simulink model "line_choices_snt"  (R2025b)
settings: Solver=ode45  StartTime=0.0  StopTime=10.0  RelTol=1e-3  EnableMultiTasking=on
values from neighbouring files (symbols this model uses):
  ft2km = 0.0003048    [IEEE_123_data.m]    (also in IEEE_123_data_fault.m)
undefined symbols (not defined in the file or in its folder): C_1, find_system, L_1, R_1
libraries: fl_lib x156, nesl_utility x24
(part 2 of 2)

== system line_choices_snt/T2sscT/OLTC ==
  Electrical Reference : fl_lib/Electrical/Electrical Elements/Electrical Reference
  Electrical Reference1 : fl_lib/Electrical/Electrical Elements/Electrical Reference
  TA : Subsystem
  TB : Subsystem
  A : PMIOPort  Tag=PMCPort  Side=Left
  B : PMIOPort  Tag=PMCPort  Port=2  Side=Left
  a : PMIOPort  Tag=PMCPort  Port=3  Side=Right
  b : PMIOPort  Tag=PMCPort  Port=4  Side=Right
  connections:
  Electrical Reference1/LConn1 -- TB/RConn2 -- TA/RConn2
  TA/RConn1 -- a/RConn1
  TA/LConn1 -- A/RConn1
  TB/LConn1 -- B/RConn1
  TB/RConn1 -- b/RConn1
  Electrical Reference/LConn1 -- TB/LConn2 -- TA/LConn2

== system line_choices_snt/T2sscT/Pi-Section Line ==
  Array Connection{,1..3} (4 alike) : SimscapeArrayConnection
  Electrical Reference : fl_lib/Electrical/Electrical Elements/Electrical Reference
  Electrical Reference1 : fl_lib/Electrical/Electrical Elements/Electrical Reference
  Mutual C1 : SimscapeComponentBlock  SourceFile=multi_coupled_C  ComponentPath=multi_coupled_C  ComponentVariants="[\"multi_coupled_C\"]"  ComponentVariantNames="[\"multi_coupled_C\"]"  ClassName=multi_coupled_C  SchemaVersion=1  noph=2  C=C F
      settings: CopyFcn=simscape.sscblock.internal.componentBlockCallback(gcbh,'COPY')  PreCopyFcn=simscape.sscblock.internal.componentBlockCallback(gcbh,'PRECOPY')  PreDeleteFcn=simscape.sscblock.internal.componentBlockCallback(gcbh,'PREDELETE')  InternalSimscapePortConfiguration="{\"Bottom\":[],\"Left\":[{\"id\":\"p\",\"label\":\"p\",\"type\":\"foundation.electrical.electrical\"}],\"Right\":[{\"id\":\"n\",\"label\":\"n\",\"type\":\"foundation.electrical.electrical\"}],\"Top\":[]}"
      mask Type: Multi-Phase Coupled C
  Mutual C2 : SimscapeComponentBlock  SourceFile=multi_coupled_C  ComponentPath=multi_coupled_C  ComponentVariants="[\"multi_coupled_C\"]"  ComponentVariantNames="[\"multi_coupled_C\"]"  ClassName=multi_coupled_C  SchemaVersion=1  noph=2  C=C F
      settings: CopyFcn=simscape.sscblock.internal.componentBlockCallback(gcbh,'COPY')  PreCopyFcn=simscape.sscblock.internal.componentBlockCallback(gcbh,'PRECOPY')  PreDeleteFcn=simscape.sscblock.internal.componentBlockCallback(gcbh,'PREDELETE')  InternalSimscapePortConfiguration="{\"Bottom\":[],\"Left\":[{\"id\":\"p\",\"label\":\"p\",\"type\":\"foundation.electrical.electrical\"}],\"Right\":[{\"id\":\"n\",\"label\":\"n\",\"type\":\"foundation.electrical.electrical\"}],\"Top\":[]}"
      mask Type: Multi-Phase Coupled C
  Mutual RL : SimscapeComponentBlock  SourceFile=multi_coupled_RL  ComponentPath=multi_coupled_RL  ComponentVariants="[\"multi_coupled_RL\"]"  ComponentVariantNames="[\"multi_coupled_RL\"]"  ClassName=multi_coupled_RL  SchemaVersion=1  noph=2  R=R Ohm  L=L H
      settings: CopyFcn=simscape.sscblock.internal.componentBlockCallback(gcbh,'COPY')  PreCopyFcn=simscape.sscblock.internal.componentBlockCallback(gcbh,'PRECOPY')  PreDeleteFcn=simscape.sscblock.internal.componentBlockCallback(gcbh,'PREDELETE')  InternalSimscapePortConfiguration="{\"Bottom\":[],\"Left\":[{\"id\":\"p\",\"label\":\"p\",\"type\":\"foundation.electrical.electrical\"}],\"Right\":[{\"id\":\"n\",\"label\":\"n\",\"type\":\"foundation.electrical.electrical\"}],\"Top\":[]}"
      mask Type: Multi-Phase Coupled RL
  PS-Simulink Converter : nesl_utility/PS-Simulink Converter  PhysicalDomain=network_engine_domain  SubClassName=ps_output  LeftPortType=input  RightPortType=output  PseudoPeriodic=off  Frequencies=[]  VectorFormat=inherit  Unit=inherit  AffineConversion=off
  Simscape Component : SimscapeComponentBlock  SourceFile=multi_current  ComponentPath=multi_current  ComponentVariants="[\"multi_current\"]"  ComponentVariantNames="[\"multi_current\"]"  ClassName=multi_current  SchemaVersion=1  noph=2
      settings: CopyFcn=simscape.sscblock.internal.componentBlockCallback(gcbh,'COPY')  PreCopyFcn=simscape.sscblock.internal.componentBlockCallback(gcbh,'PRECOPY')  PreDeleteFcn=simscape.sscblock.internal.componentBlockCallback(gcbh,'PREDELETE')  InternalSimscapePortConfiguration="{\"Bottom\":[],\"Left\":[{\"id\":\"p\",\"label\":\"+\",\"type\":\"foundation.electrical.electrical\"}],\"Right\":[{\"id\":\"I\",\"label\":\"I\",\"type\":\"output\"},{\"id\":\"n\",\"label\":\"-\",\"type\":\"foundation.electrical.electrical\"}],\"Top\":[]}"
      mask Type: Multi-Phase Current Sensor
  A : PMIOPort  Side=Left
  B : PMIOPort  Port=2  Side=Left
  a : PMIOPort  Port=3  Side=Right
  b : PMIOPort  Port=4  Side=Right
  Imeas : Outport
  wires:
  PS-Simulink Converter/1 -> Imeas/1
  connections:
  Mutual RL/RConn1 -- Array Connection1/RConn1 -- Mutual C2/LConn1
  Mutual C1/LConn1 -- Simscape Component/RConn2 -- Mutual RL/LConn1
  PS-Simulink Converter/LConn1 -- Simscape Component/RConn1
  Array Connection/RConn1 -- Simscape Component/LConn1
  A/RConn1 -- Array Connection/LConn1
  B/RConn1 -- Array Connection/LConn2
  a/RConn1 -- Array Connection1/LConn1
  b/RConn1 -- Array Connection1/LConn2
  Array Connection2/RConn1 -- Mutual C1/RConn1
  Array Connection3/RConn1 -- Mutual C2/RConn1
  Array Connection2/LConn1 -- Electrical Reference/LConn1 -- Array Connection2/LConn2
  Array Connection3/LConn1 -- Electrical Reference1/LConn1 -- Array Connection3/LConn2

== system line_choices_snt/T2sscTf/OLTC ==
  Electrical Reference : fl_lib/Electrical/Electrical Elements/Electrical Reference
  Electrical Reference1 : fl_lib/Electrical/Electrical Elements/Electrical Reference
  TA : Subsystem
  TB : Subsystem
  A : PMIOPort  Tag=PMCPort  Side=Left
  B : PMIOPort  Tag=PMCPort  Port=2  Side=Left
  a : PMIOPort  Tag=PMCPort  Port=3  Side=Right
  b : PMIOPort  Tag=PMCPort  Port=4  Side=Right
  connections:
  TA/LConn2 -- TB/LConn2 -- Electrical Reference/LConn1
  TB/RConn1 -- b/RConn1
  TB/LConn1 -- B/RConn1
  TA/LConn1 -- A/RConn1
  TA/RConn1 -- a/RConn1
  TA/RConn2 -- TB/RConn2 -- Electrical Reference1/LConn1

== system line_choices_snt/T2sscTf/Pi-Section Line ==
  Array Connection{,1..3} (4 alike) : SimscapeArrayConnection
  Electrical Reference : fl_lib/Electrical/Electrical Elements/Electrical Reference
  Electrical Reference1 : fl_lib/Electrical/Electrical Elements/Electrical Reference
  Mutual C1 : SimscapeComponentBlock  SourceFile=multi_coupled_C  ComponentPath=multi_coupled_C  ComponentVariants="[\"multi_coupled_C\"]"  ComponentVariantNames="[\"multi_coupled_C\"]"  ClassName=multi_coupled_C  SchemaVersion=1  noph=2  C=C F
      settings: CopyFcn=simscape.sscblock.internal.componentBlockCallback(gcbh,'COPY')  PreCopyFcn=simscape.sscblock.internal.componentBlockCallback(gcbh,'PRECOPY')  PreDeleteFcn=simscape.sscblock.internal.componentBlockCallback(gcbh,'PREDELETE')  InternalSimscapePortConfiguration="{\"Bottom\":[],\"Left\":[{\"id\":\"p\",\"label\":\"p\",\"type\":\"foundation.electrical.electrical\"}],\"Right\":[{\"id\":\"n\",\"label\":\"n\",\"type\":\"foundation.electrical.electrical\"}],\"Top\":[]}"
      mask Type: Multi-Phase Coupled C
  Mutual C2 : SimscapeComponentBlock  SourceFile=multi_coupled_C  ComponentPath=multi_coupled_C  ComponentVariants="[\"multi_coupled_C\"]"  ComponentVariantNames="[\"multi_coupled_C\"]"  ClassName=multi_coupled_C  SchemaVersion=1  noph=2  C=C F
      settings: CopyFcn=simscape.sscblock.internal.componentBlockCallback(gcbh,'COPY')  PreCopyFcn=simscape.sscblock.internal.componentBlockCallback(gcbh,'PRECOPY')  PreDeleteFcn=simscape.sscblock.internal.componentBlockCallback(gcbh,'PREDELETE')  InternalSimscapePortConfiguration="{\"Bottom\":[],\"Left\":[{\"id\":\"p\",\"label\":\"p\",\"type\":\"foundation.electrical.electrical\"}],\"Right\":[{\"id\":\"n\",\"label\":\"n\",\"type\":\"foundation.electrical.electrical\"}],\"Top\":[]}"
      mask Type: Multi-Phase Coupled C
  Mutual RL : SimscapeComponentBlock  SourceFile=multi_coupled_RL  ComponentPath=multi_coupled_RL  ComponentVariants="[\"multi_coupled_RL\"]"  ComponentVariantNames="[\"multi_coupled_RL\"]"  ClassName=multi_coupled_RL  SchemaVersion=1  noph=2  R=R Ohm  L=L H
      settings: CopyFcn=simscape.sscblock.internal.componentBlockCallback(gcbh,'COPY')  PreCopyFcn=simscape.sscblock.internal.componentBlockCallback(gcbh,'PRECOPY')  PreDeleteFcn=simscape.sscblock.internal.componentBlockCallback(gcbh,'PREDELETE')  InternalSimscapePortConfiguration="{\"Bottom\":[],\"Left\":[{\"id\":\"p\",\"label\":\"p\",\"type\":\"foundation.electrical.electrical\"}],\"Right\":[{\"id\":\"n\",\"label\":\"n\",\"type\":\"foundation.electrical.electrical\"}],\"Top\":[]}"
      mask Type: Multi-Phase Coupled RL
  PS-Simulink Converter : nesl_utility/PS-Simulink Converter  PhysicalDomain=network_engine_domain  SubClassName=ps_output  LeftPortType=input  RightPortType=output  PseudoPeriodic=off  Frequencies=[]  VectorFormat=inherit  Unit=inherit  AffineConversion=off
  Simscape Component : SimscapeComponentBlock  SourceFile=multi_current  ComponentPath=multi_current  ComponentVariants="[\"multi_current\"]"  ComponentVariantNames="[\"multi_current\"]"  ClassName=multi_current  SchemaVersion=1  noph=2
      settings: CopyFcn=simscape.sscblock.internal.componentBlockCallback(gcbh,'COPY')  PreCopyFcn=simscape.sscblock.internal.componentBlockCallback(gcbh,'PRECOPY')  PreDeleteFcn=simscape.sscblock.internal.componentBlockCallback(gcbh,'PREDELETE')  InternalSimscapePortConfiguration="{\"Bottom\":[],\"Left\":[{\"id\":\"p\",\"label\":\"+\",\"type\":\"foundation.electrical.electrical\"}],\"Right\":[{\"id\":\"I\",\"label\":\"I\",\"type\":\"output\"},{\"id\":\"n\",\"label\":\"-\",\"type\":\"foundation.electrical.electrical\"}],\"Top\":[]}"
      mask Type: Multi-Phase Current Sensor
  A : PMIOPort  Side=Left
  B : PMIOPort  Port=2  Side=Left
  a : PMIOPort  Port=3  Side=Right
  b : PMIOPort  Port=4  Side=Right
  Imeas : Outport
  wires:
  PS-Simulink Converter/1 -> Imeas/1
  connections:
  Array Connection3/LConn2 -- Electrical Reference1/LConn1 -- Array Connection3/LConn1
  Array Connection2/LConn2 -- Electrical Reference/LConn1 -- Array Connection2/LConn1
  Array Connection3/RConn1 -- Mutual C2/RConn1
  Array Connection2/RConn1 -- Mutual C1/RConn1
  b/RConn1 -- Array Connection1/LConn2
  a/RConn1 -- Array Connection1/LConn1
  B/RConn1 -- Array Connection/LConn2
  A/RConn1 -- Array Connection/LConn1
  Array Connection/RConn1 -- Simscape Component/LConn1
  PS-Simulink Converter/LConn1 -- Simscape Component/RConn1
  Mutual RL/LConn1 -- Simscape Component/RConn2 -- Mutual C1/LConn1
  Mutual C2/LConn1 -- Array Connection1/RConn1 -- Mutual RL/RConn1

== system line_choices_snt/T3sscT/OLTC ==
  Electrical Reference : fl_lib/Electrical/Electrical Elements/Electrical Reference
  Electrical Reference1 : fl_lib/Electrical/Electrical Elements/Electrical Reference
  TA : Subsystem
  TB : Subsystem
  TC : Subsystem
  A : PMIOPort  Tag=PMCPort  Side=Left
  B : PMIOPort  Tag=PMCPort  Port=2  Side=Left
  C : PMIOPort  Tag=PMCPort  Port=3  Side=Left
  a : PMIOPort  Tag=PMCPort  Port=4  Side=Right
  b : PMIOPort  Tag=PMCPort  Port=5  Side=Right
  c : PMIOPort  Tag=PMCPort  Port=6  Side=Right
  connections:
  TA/RConn1 -- a/RConn1
  TA/LConn1 -- A/RConn1
  TB/LConn1 -- B/RConn1
  TB/RConn1 -- b/RConn1
  TC/LConn1 -- C/RConn1
  TC/RConn1 -- c/RConn1
  TB/RConn2 -- TA/RConn2 -- TC/RConn2 -- Electrical Reference1/LConn1
  TB/LConn2 -- TA/LConn2 -- TC/LConn2 -- Electrical Reference/LConn1

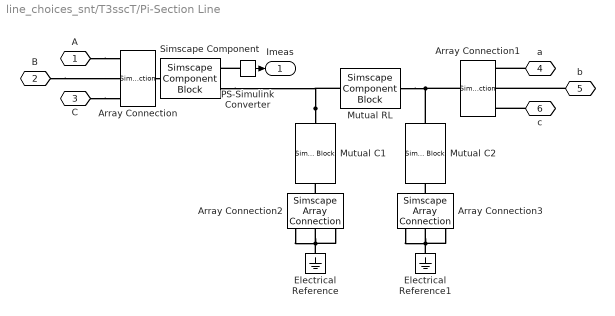
== system line_choices_snt/T3sscT/Pi-Section Line ==
  Array Connection{,1..3} (4 alike) : SimscapeArrayConnection  NumScalarElements=3
  Electrical Reference : fl_lib/Electrical/Electrical Elements/Electrical Reference
  Electrical Reference1 : fl_lib/Electrical/Electrical Elements/Electrical Reference
  Mutual C1 : SimscapeComponentBlock  SourceFile=multi_coupled_C  ComponentPath=multi_coupled_C  ComponentVariants="[\"multi_coupled_C\"]"  ComponentVariantNames="[\"multi_coupled_C\"]"  ClassName=multi_coupled_C  SchemaVersion=1  noph=3  C=C F
      settings: CopyFcn=simscape.sscblock.internal.componentBlockCallback(gcbh,'COPY')  PreCopyFcn=simscape.sscblock.internal.componentBlockCallback(gcbh,'PRECOPY')  PreDeleteFcn=simscape.sscblock.internal.componentBlockCallback(gcbh,'PREDELETE')  InternalSimscapePortConfiguration="{\"Bottom\":[],\"Left\":[{\"id\":\"p\",\"label\":\"p\",\"type\":\"foundation.electrical.electrical\"}],\"Right\":[{\"id\":\"n\",\"label\":\"n\",\"type\":\"foundation.electrical.electrical\"}],\"Top\":[]}"
      mask Type: Multi-Phase Coupled C
  Mutual C2 : SimscapeComponentBlock  SourceFile=multi_coupled_C  ComponentPath=multi_coupled_C  ComponentVariants="[\"multi_coupled_C\"]"  ComponentVariantNames="[\"multi_coupled_C\"]"  ClassName=multi_coupled_C  SchemaVersion=1  noph=3  C=C F
      settings: CopyFcn=simscape.sscblock.internal.componentBlockCallback(gcbh,'COPY')  PreCopyFcn=simscape.sscblock.internal.componentBlockCallback(gcbh,'PRECOPY')  PreDeleteFcn=simscape.sscblock.internal.componentBlockCallback(gcbh,'PREDELETE')  InternalSimscapePortConfiguration="{\"Bottom\":[],\"Left\":[{\"id\":\"p\",\"label\":\"p\",\"type\":\"foundation.electrical.electrical\"}],\"Right\":[{\"id\":\"n\",\"label\":\"n\",\"type\":\"foundation.electrical.electrical\"}],\"Top\":[]}"
      mask Type: Multi-Phase Coupled C
  Mutual RL : SimscapeComponentBlock  SourceFile=multi_coupled_RL  ComponentPath=multi_coupled_RL  ComponentVariants="[\"multi_coupled_RL\"]"  ComponentVariantNames="[\"multi_coupled_RL\"]"  ClassName=multi_coupled_RL  SchemaVersion=1  noph=3  R=R Ohm  L=L H
      settings: CopyFcn=simscape.sscblock.internal.componentBlockCallback(gcbh,'COPY')  PreCopyFcn=simscape.sscblock.internal.componentBlockCallback(gcbh,'PRECOPY')  PreDeleteFcn=simscape.sscblock.internal.componentBlockCallback(gcbh,'PREDELETE')  InternalSimscapePortConfiguration="{\"Bottom\":[],\"Left\":[{\"id\":\"p\",\"label\":\"p\",\"type\":\"foundation.electrical.electrical\"}],\"Right\":[{\"id\":\"n\",\"label\":\"n\",\"type\":\"foundation.electrical.electrical\"}],\"Top\":[]}"
      mask Type: Multi-Phase Coupled RL
  PS-Simulink Converter : nesl_utility/PS-Simulink Converter  PhysicalDomain=network_engine_domain  SubClassName=ps_output  LeftPortType=input  RightPortType=output  PseudoPeriodic=off  Frequencies=[]  VectorFormat=inherit  Unit=inherit  AffineConversion=off
  Simscape Component : SimscapeComponentBlock  SourceFile=multi_current  ComponentPath=multi_current  ComponentVariants="[\"multi_current\"]"  ComponentVariantNames="[\"multi_current\"]"  ClassName=multi_current  SchemaVersion=1  noph=3
      settings: CopyFcn=simscape.sscblock.internal.componentBlockCallback(gcbh,'COPY')  PreCopyFcn=simscape.sscblock.internal.componentBlockCallback(gcbh,'PRECOPY')  PreDeleteFcn=simscape.sscblock.internal.componentBlockCallback(gcbh,'PREDELETE')  InternalSimscapePortConfiguration="{\"Bottom\":[],\"Left\":[{\"id\":\"p\",\"label\":\"+\",\"type\":\"foundation.electrical.electrical\"}],\"Right\":[{\"id\":\"I\",\"label\":\"I\",\"type\":\"output\"},{\"id\":\"n\",\"label\":\"-\",\"type\":\"foundation.electrical.electrical\"}],\"Top\":[]}"
      mask Type: Multi-Phase Current Sensor
  A : PMIOPort  Side=Left
  B : PMIOPort  Port=2  Side=Left
  C : PMIOPort  Port=3  Side=Left
  a : PMIOPort  Port=4  Side=Right
  b : PMIOPort  Port=5  Side=Right
  c : PMIOPort  Port=6  Side=Right
  Imeas : Outport
  wires:
  PS-Simulink Converter/1 -> Imeas/1
  connections:
  Array Connection2/LConn2 -- Array Connection2/LConn3 -- Array Connection2/LConn1 -- Electrical Reference/LConn1
  Mutual RL/RConn1 -- Array Connection1/RConn1 -- Mutual C2/LConn1
  Mutual C1/LConn1 -- Simscape Component/RConn2 -- Mutual RL/LConn1
  Array Connection3/LConn1 -- Array Connection3/LConn2 -- Array Connection3/LConn3 -- Electrical Reference1/LConn1
  Array Connection2/RConn1 -- Mutual C1/RConn1
  Array Connection/RConn1 -- Simscape Component/LConn1
  PS-Simulink Converter/LConn1 -- Simscape Component/RConn1
  Array Connection3/RConn1 -- Mutual C2/RConn1
  A/RConn1 -- Array Connection/LConn1
  B/RConn1 -- Array Connection/LConn2
  C/RConn1 -- Array Connection/LConn3
  a/RConn1 -- Array Connection1/LConn1
  b/RConn1 -- Array Connection1/LConn2
  c/RConn1 -- Array Connection1/LConn3

== system line_choices_snt/T3sscTf/OLTC ==
  Electrical Reference : fl_lib/Electrical/Electrical Elements/Electrical Reference
  Electrical Reference1 : fl_lib/Electrical/Electrical Elements/Electrical Reference
  TA : Subsystem
  TB : Subsystem
  TC : Subsystem
  A : PMIOPort  Tag=PMCPort  Side=Left
  B : PMIOPort  Tag=PMCPort  Port=2  Side=Left
  C : PMIOPort  Tag=PMCPort  Port=3  Side=Left
  a : PMIOPort  Tag=PMCPort  Port=4  Side=Right
  b : PMIOPort  Tag=PMCPort  Port=5  Side=Right
  c : PMIOPort  Tag=PMCPort  Port=6  Side=Right
  connections:
  Electrical Reference/LConn1 -- TC/LConn2 -- TA/LConn2 -- TB/LConn2
  Electrical Reference1/LConn1 -- TC/RConn2 -- TA/RConn2 -- TB/RConn2
  TC/RConn1 -- c/RConn1
  TC/LConn1 -- C/RConn1
  TB/RConn1 -- b/RConn1
  TB/LConn1 -- B/RConn1
  TA/LConn1 -- A/RConn1
  TA/RConn1 -- a/RConn1

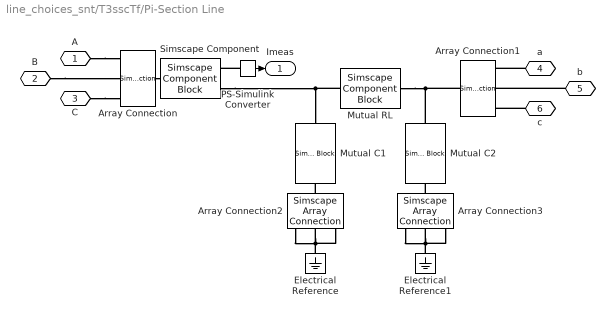
== system line_choices_snt/T3sscTf/Pi-Section Line ==
  Array Connection{,1..3} (4 alike) : SimscapeArrayConnection  NumScalarElements=3
  Electrical Reference : fl_lib/Electrical/Electrical Elements/Electrical Reference
  Electrical Reference1 : fl_lib/Electrical/Electrical Elements/Electrical Reference
  Mutual C1 : SimscapeComponentBlock  SourceFile=multi_coupled_C  ComponentPath=multi_coupled_C  ComponentVariants="[\"multi_coupled_C\"]"  ComponentVariantNames="[\"multi_coupled_C\"]"  ClassName=multi_coupled_C  SchemaVersion=1  noph=3  C=C F
      settings: CopyFcn=simscape.sscblock.internal.componentBlockCallback(gcbh,'COPY')  PreCopyFcn=simscape.sscblock.internal.componentBlockCallback(gcbh,'PRECOPY')  PreDeleteFcn=simscape.sscblock.internal.componentBlockCallback(gcbh,'PREDELETE')  InternalSimscapePortConfiguration="{\"Bottom\":[],\"Left\":[{\"id\":\"p\",\"label\":\"p\",\"type\":\"foundation.electrical.electrical\"}],\"Right\":[{\"id\":\"n\",\"label\":\"n\",\"type\":\"foundation.electrical.electrical\"}],\"Top\":[]}"
      mask Type: Multi-Phase Coupled C
  Mutual C2 : SimscapeComponentBlock  SourceFile=multi_coupled_C  ComponentPath=multi_coupled_C  ComponentVariants="[\"multi_coupled_C\"]"  ComponentVariantNames="[\"multi_coupled_C\"]"  ClassName=multi_coupled_C  SchemaVersion=1  noph=3  C=C F
      settings: CopyFcn=simscape.sscblock.internal.componentBlockCallback(gcbh,'COPY')  PreCopyFcn=simscape.sscblock.internal.componentBlockCallback(gcbh,'PRECOPY')  PreDeleteFcn=simscape.sscblock.internal.componentBlockCallback(gcbh,'PREDELETE')  InternalSimscapePortConfiguration="{\"Bottom\":[],\"Left\":[{\"id\":\"p\",\"label\":\"p\",\"type\":\"foundation.electrical.electrical\"}],\"Right\":[{\"id\":\"n\",\"label\":\"n\",\"type\":\"foundation.electrical.electrical\"}],\"Top\":[]}"
      mask Type: Multi-Phase Coupled C
  Mutual RL : SimscapeComponentBlock  SourceFile=multi_coupled_RL  ComponentPath=multi_coupled_RL  ComponentVariants="[\"multi_coupled_RL\"]"  ComponentVariantNames="[\"multi_coupled_RL\"]"  ClassName=multi_coupled_RL  SchemaVersion=1  noph=3  R=R Ohm  L=L H
      settings: CopyFcn=simscape.sscblock.internal.componentBlockCallback(gcbh,'COPY')  PreCopyFcn=simscape.sscblock.internal.componentBlockCallback(gcbh,'PRECOPY')  PreDeleteFcn=simscape.sscblock.internal.componentBlockCallback(gcbh,'PREDELETE')  InternalSimscapePortConfiguration="{\"Bottom\":[],\"Left\":[{\"id\":\"p\",\"label\":\"p\",\"type\":\"foundation.electrical.electrical\"}],\"Right\":[{\"id\":\"n\",\"label\":\"n\",\"type\":\"foundation.electrical.electrical\"}],\"Top\":[]}"
      mask Type: Multi-Phase Coupled RL
  PS-Simulink Converter : nesl_utility/PS-Simulink Converter  PhysicalDomain=network_engine_domain  SubClassName=ps_output  LeftPortType=input  RightPortType=output  PseudoPeriodic=off  Frequencies=[]  VectorFormat=inherit  Unit=inherit  AffineConversion=off
  Simscape Component : SimscapeComponentBlock  SourceFile=multi_current  ComponentPath=multi_current  ComponentVariants="[\"multi_current\"]"  ComponentVariantNames="[\"multi_current\"]"  ClassName=multi_current  SchemaVersion=1  noph=3
      settings: CopyFcn=simscape.sscblock.internal.componentBlockCallback(gcbh,'COPY')  PreCopyFcn=simscape.sscblock.internal.componentBlockCallback(gcbh,'PRECOPY')  PreDeleteFcn=simscape.sscblock.internal.componentBlockCallback(gcbh,'PREDELETE')  InternalSimscapePortConfiguration="{\"Bottom\":[],\"Left\":[{\"id\":\"p\",\"label\":\"+\",\"type\":\"foundation.electrical.electrical\"}],\"Right\":[{\"id\":\"I\",\"label\":\"I\",\"type\":\"output\"},{\"id\":\"n\",\"label\":\"-\",\"type\":\"foundation.electrical.electrical\"}],\"Top\":[]}"
      mask Type: Multi-Phase Current Sensor
  A : PMIOPort  Side=Left
  B : PMIOPort  Port=2  Side=Left
  C : PMIOPort  Port=3  Side=Left
  a : PMIOPort  Port=4  Side=Right
  b : PMIOPort  Port=5  Side=Right
  c : PMIOPort  Port=6  Side=Right
  Imeas : Outport
  wires:
  PS-Simulink Converter/1 -> Imeas/1
  connections:
  c/RConn1 -- Array Connection1/LConn3
  b/RConn1 -- Array Connection1/LConn2
  a/RConn1 -- Array Connection1/LConn1
  C/RConn1 -- Array Connection/LConn3
  B/RConn1 -- Array Connection/LConn2
  A/RConn1 -- Array Connection/LConn1
  Array Connection3/RConn1 -- Mutual C2/RConn1
  PS-Simulink Converter/LConn1 -- Simscape Component/RConn1
  Array Connection/RConn1 -- Simscape Component/LConn1
  Array Connection2/RConn1 -- Mutual C1/RConn1
  Electrical Reference1/LConn1 -- Array Connection3/LConn3 -- Array Connection3/LConn2 -- Array Connection3/LConn1
  Mutual RL/LConn1 -- Simscape Component/RConn2 -- Mutual C1/LConn1
  Mutual C2/LConn1 -- Array Connection1/RConn1 -- Mutual RL/RConn1
  Electrical Reference/LConn1 -- Array Connection2/LConn1 -- Array Connection2/LConn3 -- Array Connection2/LConn2

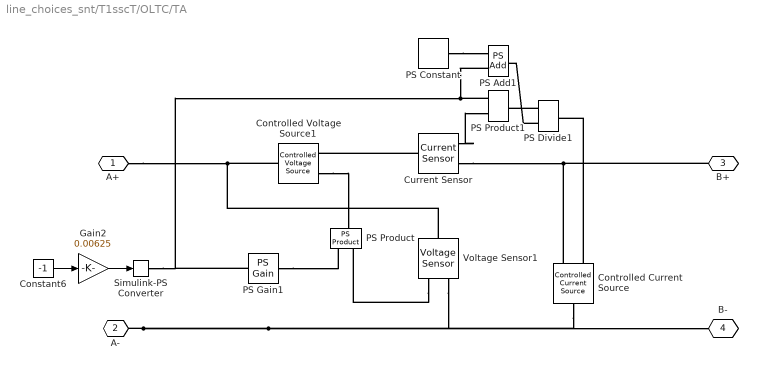
== system line_choices_snt/T1sscT/OLTC/TA ==
  Constant6 : Constant  Value=-1
  Controlled Current Source : fl_lib/Electrical/Electrical Sources/Controlled Current Source
  Controlled Voltage Source1 : fl_lib/Electrical/Electrical Sources/Controlled Voltage Source
  Current Sensor : fl_lib/Electrical/Electrical Sensors/Current Sensor
  Gain2 : Gain  Gain=0.00625
  PS Add1 : fl_lib/Physical Signals/Functions/PS Add
  PS Constant : fl_lib/Physical Signals/Sources/PS Constant  constant=1
  PS Divide1 : fl_lib/Physical Signals/Functions/PS Divide
  PS Gain1 : fl_lib/Physical Signals/Functions/PS Gain  gain=-1
  PS Product : fl_lib/Physical Signals/Functions/PS Product
  PS Product1 : fl_lib/Physical Signals/Functions/PS Product
  Simulink-PS Converter : nesl_utility/Simulink-PS Converter  PhysicalDomain=network_engine_domain  SubClassName=ps_input  LeftPortType=input  RightPortType=output  PseudoPeriodic=off  Frequencies=[]  NoiseDistribution=none  NoiseParameters=[]  Unit=1  AffineConversion=off  FilteringAndDerivatives=zero  SimscapeFilterOrder=1  InputFilterTimeConstant=0.001  UdotUserProvided=0
  Voltage Sensor1 : fl_lib/Electrical/Electrical Sensors/Voltage Sensor
  A+ : PMIOPort  Side=Left
  A- : PMIOPort  Port=2  Side=Left
  B+ : PMIOPort  Port=3  Side=Right
  B- : PMIOPort  Port=4  Side=Right
  wires:
  Gain2/1 -> Simulink-PS Converter/1
  Constant6/1 -> Gain2/1
  connections:
  PS Constant/RConn1 -- PS Add1/LConn1
  PS Divide1/LConn2 -- PS Add1/RConn1
  PS Divide1/LConn1 -- PS Product1/RConn1
  PS Gain1/LConn1 -- Simulink-PS Converter/RConn1 -- PS Add1/LConn2 -- PS Product1/LConn1
  PS Gain1/RConn1 -- PS Product/LConn1
  Voltage Sensor1/RConn1 -- PS Product/LConn2
  A+/RConn1 -- Voltage Sensor1/LConn1 -- Controlled Voltage Source1/LConn1
  Current Sensor/LConn1 -- Controlled Voltage Source1/RConn2
  B+/RConn1 -- Current Sensor/RConn2 -- Controlled Current Source/RConn2
  A-/RConn1 -- Voltage Sensor1/RConn2 -- Controlled Current Source/LConn1 -- B-/RConn1
  Controlled Voltage Source1/RConn1 -- PS Product/RConn1
  Current Sensor/RConn1 -- PS Product1/LConn2
  Controlled Current Source/RConn1 -- PS Divide1/RConn1

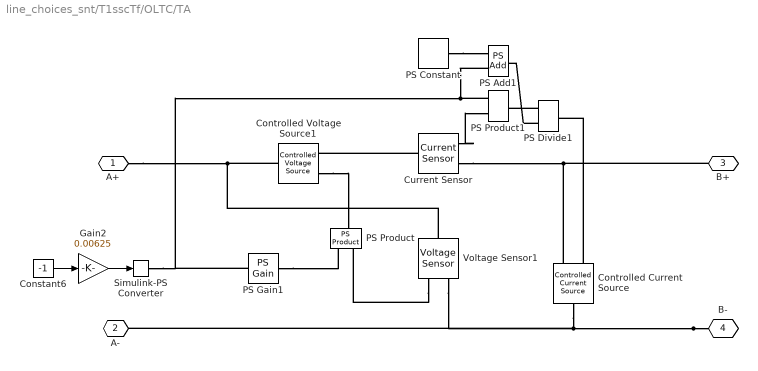
== system line_choices_snt/T1sscTf/OLTC/TA ==
  Constant6 : Constant  Value=-1
  Controlled Current Source : fl_lib/Electrical/Electrical Sources/Controlled Current Source
  Controlled Voltage Source1 : fl_lib/Electrical/Electrical Sources/Controlled Voltage Source
  Current Sensor : fl_lib/Electrical/Electrical Sensors/Current Sensor
  Gain2 : Gain  Gain=0.00625
  PS Add1 : fl_lib/Physical Signals/Functions/PS Add
  PS Constant : fl_lib/Physical Signals/Sources/PS Constant  constant=1
  PS Divide1 : fl_lib/Physical Signals/Functions/PS Divide
  PS Gain1 : fl_lib/Physical Signals/Functions/PS Gain  gain=-1
  PS Product : fl_lib/Physical Signals/Functions/PS Product
  PS Product1 : fl_lib/Physical Signals/Functions/PS Product
  Simulink-PS Converter : nesl_utility/Simulink-PS Converter  PhysicalDomain=network_engine_domain  SubClassName=ps_input  LeftPortType=input  RightPortType=output  PseudoPeriodic=off  Frequencies=[]  NoiseDistribution=none  NoiseParameters=[]  Unit=1  AffineConversion=off  FilteringAndDerivatives=zero  SimscapeFilterOrder=1  InputFilterTimeConstant=0.001  UdotUserProvided=0
  Voltage Sensor1 : fl_lib/Electrical/Electrical Sensors/Voltage Sensor
  A+ : PMIOPort  Side=Left
  A- : PMIOPort  Port=2  Side=Left
  B+ : PMIOPort  Port=3  Side=Right
  B- : PMIOPort  Port=4  Side=Right
  wires:
  Constant6/1 -> Gain2/1
  Gain2/1 -> Simulink-PS Converter/1
  connections:
  Controlled Current Source/RConn1 -- PS Divide1/RConn1
  Current Sensor/RConn1 -- PS Product1/LConn2
  Controlled Voltage Source1/RConn1 -- PS Product/RConn1
  B-/RConn1 -- Controlled Current Source/LConn1 -- Voltage Sensor1/RConn2 -- A-/RConn1
  Controlled Current Source/RConn2 -- Current Sensor/RConn2 -- B+/RConn1
  Current Sensor/LConn1 -- Controlled Voltage Source1/RConn2
  Controlled Voltage Source1/LConn1 -- Voltage Sensor1/LConn1 -- A+/RConn1
  Voltage Sensor1/RConn1 -- PS Product/LConn2
  PS Gain1/RConn1 -- PS Product/LConn1
  PS Product1/LConn1 -- PS Add1/LConn2 -- Simulink-PS Converter/RConn1 -- PS Gain1/LConn1
  PS Divide1/LConn1 -- PS Product1/RConn1
  PS Divide1/LConn2 -- PS Add1/RConn1
  PS Constant/RConn1 -- PS Add1/LConn1

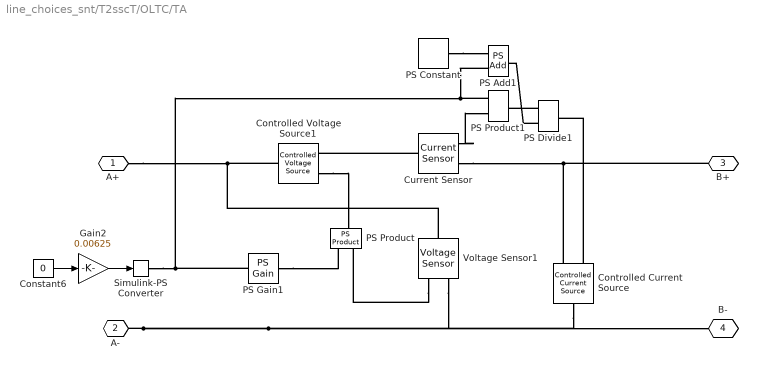
== system line_choices_snt/T2sscT/OLTC/TA ==
  Constant6 : Constant  Value=0
  Controlled Current Source : fl_lib/Electrical/Electrical Sources/Controlled Current Source
  Controlled Voltage Source1 : fl_lib/Electrical/Electrical Sources/Controlled Voltage Source
  Current Sensor : fl_lib/Electrical/Electrical Sensors/Current Sensor
  Gain2 : Gain  Gain=0.00625
  PS Add1 : fl_lib/Physical Signals/Functions/PS Add
  PS Constant : fl_lib/Physical Signals/Sources/PS Constant  constant=1
  PS Divide1 : fl_lib/Physical Signals/Functions/PS Divide
  PS Gain1 : fl_lib/Physical Signals/Functions/PS Gain  gain=-1
  PS Product : fl_lib/Physical Signals/Functions/PS Product
  PS Product1 : fl_lib/Physical Signals/Functions/PS Product
  Simulink-PS Converter : nesl_utility/Simulink-PS Converter  PhysicalDomain=network_engine_domain  SubClassName=ps_input  LeftPortType=input  RightPortType=output  PseudoPeriodic=off  Frequencies=[]  NoiseDistribution=none  NoiseParameters=[]  Unit=1  AffineConversion=off  FilteringAndDerivatives=zero  SimscapeFilterOrder=1  InputFilterTimeConstant=0.001  UdotUserProvided=0
  Voltage Sensor1 : fl_lib/Electrical/Electrical Sensors/Voltage Sensor
  A+ : PMIOPort  Side=Left
  A- : PMIOPort  Port=2  Side=Left
  B+ : PMIOPort  Port=3  Side=Right
  B- : PMIOPort  Port=4  Side=Right
  wires:
  Gain2/1 -> Simulink-PS Converter/1
  Constant6/1 -> Gain2/1
  connections:
  PS Constant/RConn1 -- PS Add1/LConn1
  PS Divide1/LConn2 -- PS Add1/RConn1
  PS Divide1/LConn1 -- PS Product1/RConn1
  Simulink-PS Converter/RConn1 -- PS Add1/LConn2 -- PS Product1/LConn1 -- PS Gain1/LConn1
  PS Gain1/RConn1 -- PS Product/LConn1
  Voltage Sensor1/RConn1 -- PS Product/LConn2
  A+/RConn1 -- Controlled Voltage Source1/LConn1 -- Voltage Sensor1/LConn1
  Current Sensor/LConn1 -- Controlled Voltage Source1/RConn2
  Controlled Current Source/RConn2 -- B+/RConn1 -- Current Sensor/RConn2
  A-/RConn1 -- Controlled Current Source/LConn1 -- B-/RConn1 -- Voltage Sensor1/RConn2
  Controlled Voltage Source1/RConn1 -- PS Product/RConn1
  Current Sensor/RConn1 -- PS Product1/LConn2
  Controlled Current Source/RConn1 -- PS Divide1/RConn1

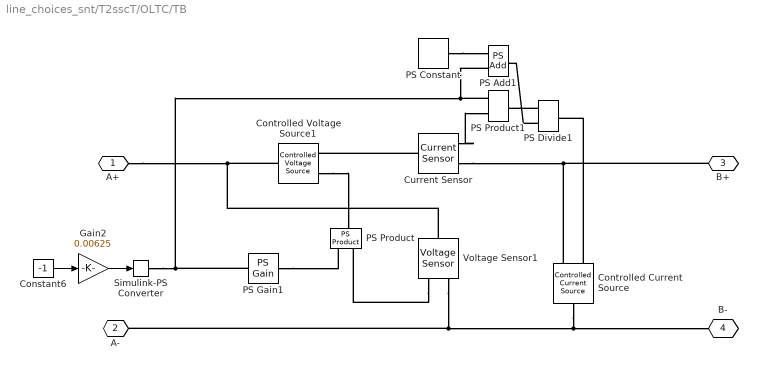
== system line_choices_snt/T2sscT/OLTC/TB ==
  Constant6 : Constant  Value=-1
  Controlled Current Source : fl_lib/Electrical/Electrical Sources/Controlled Current Source
  Controlled Voltage Source1 : fl_lib/Electrical/Electrical Sources/Controlled Voltage Source
  Current Sensor : fl_lib/Electrical/Electrical Sensors/Current Sensor
  Gain2 : Gain  Gain=0.00625
  PS Add1 : fl_lib/Physical Signals/Functions/PS Add
  PS Constant : fl_lib/Physical Signals/Sources/PS Constant  constant=1
  PS Divide1 : fl_lib/Physical Signals/Functions/PS Divide
  PS Gain1 : fl_lib/Physical Signals/Functions/PS Gain  gain=-1
  PS Product : fl_lib/Physical Signals/Functions/PS Product
  PS Product1 : fl_lib/Physical Signals/Functions/PS Product
  Simulink-PS Converter : nesl_utility/Simulink-PS Converter  PhysicalDomain=network_engine_domain  SubClassName=ps_input  LeftPortType=input  RightPortType=output  PseudoPeriodic=off  Frequencies=[]  NoiseDistribution=none  NoiseParameters=[]  Unit=1  AffineConversion=off  FilteringAndDerivatives=zero  SimscapeFilterOrder=1  InputFilterTimeConstant=0.001  UdotUserProvided=0
  Voltage Sensor1 : fl_lib/Electrical/Electrical Sensors/Voltage Sensor
  A+ : PMIOPort  Side=Left
  A- : PMIOPort  Port=2  Side=Left
  B+ : PMIOPort  Port=3  Side=Right
  B- : PMIOPort  Port=4  Side=Right
  wires:
  Constant6/1 -> Gain2/1
  Gain2/1 -> Simulink-PS Converter/1
  connections:
  Controlled Current Source/RConn1 -- PS Divide1/RConn1
  Current Sensor/RConn1 -- PS Product1/LConn2
  Controlled Voltage Source1/RConn1 -- PS Product/RConn1
  Voltage Sensor1/RConn2 -- B-/RConn1 -- Controlled Current Source/LConn1 -- A-/RConn1
  Current Sensor/RConn2 -- B+/RConn1 -- Controlled Current Source/RConn2
  Current Sensor/LConn1 -- Controlled Voltage Source1/RConn2
  Voltage Sensor1/LConn1 -- Controlled Voltage Source1/LConn1 -- A+/RConn1
  Voltage Sensor1/RConn1 -- PS Product/LConn2
  PS Gain1/RConn1 -- PS Product/LConn1
  PS Gain1/LConn1 -- PS Product1/LConn1 -- PS Add1/LConn2 -- Simulink-PS Converter/RConn1
  PS Divide1/LConn1 -- PS Product1/RConn1
  PS Divide1/LConn2 -- PS Add1/RConn1
  PS Constant/RConn1 -- PS Add1/LConn1

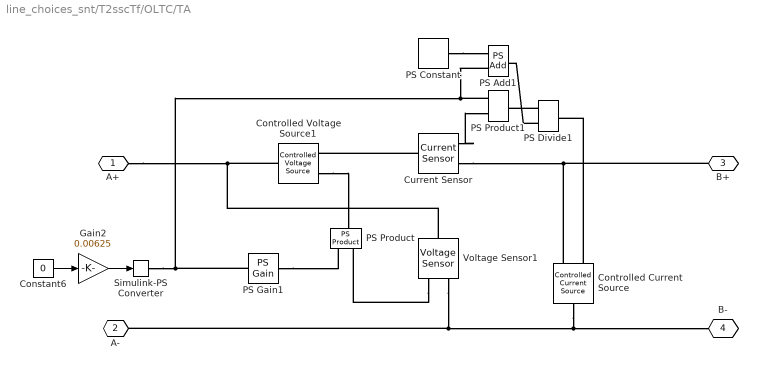
== system line_choices_snt/T2sscTf/OLTC/TA ==
  Constant6 : Constant  Value=0
  Controlled Current Source : fl_lib/Electrical/Electrical Sources/Controlled Current Source
  Controlled Voltage Source1 : fl_lib/Electrical/Electrical Sources/Controlled Voltage Source
  Current Sensor : fl_lib/Electrical/Electrical Sensors/Current Sensor
  Gain2 : Gain  Gain=0.00625
  PS Add1 : fl_lib/Physical Signals/Functions/PS Add
  PS Constant : fl_lib/Physical Signals/Sources/PS Constant  constant=1
  PS Divide1 : fl_lib/Physical Signals/Functions/PS Divide
  PS Gain1 : fl_lib/Physical Signals/Functions/PS Gain  gain=-1
  PS Product : fl_lib/Physical Signals/Functions/PS Product
  PS Product1 : fl_lib/Physical Signals/Functions/PS Product
  Simulink-PS Converter : nesl_utility/Simulink-PS Converter  PhysicalDomain=network_engine_domain  SubClassName=ps_input  LeftPortType=input  RightPortType=output  PseudoPeriodic=off  Frequencies=[]  NoiseDistribution=none  NoiseParameters=[]  Unit=1  AffineConversion=off  FilteringAndDerivatives=zero  SimscapeFilterOrder=1  InputFilterTimeConstant=0.001  UdotUserProvided=0
  Voltage Sensor1 : fl_lib/Electrical/Electrical Sensors/Voltage Sensor
  A+ : PMIOPort  Side=Left
  A- : PMIOPort  Port=2  Side=Left
  B+ : PMIOPort  Port=3  Side=Right
  B- : PMIOPort  Port=4  Side=Right
  wires:
  Constant6/1 -> Gain2/1
  Gain2/1 -> Simulink-PS Converter/1
  connections:
  Controlled Current Source/RConn1 -- PS Divide1/RConn1
  Current Sensor/RConn1 -- PS Product1/LConn2
  Controlled Voltage Source1/RConn1 -- PS Product/RConn1
  Voltage Sensor1/RConn2 -- B-/RConn1 -- Controlled Current Source/LConn1 -- A-/RConn1
  Current Sensor/RConn2 -- B+/RConn1 -- Controlled Current Source/RConn2
  Current Sensor/LConn1 -- Controlled Voltage Source1/RConn2
  Voltage Sensor1/LConn1 -- Controlled Voltage Source1/LConn1 -- A+/RConn1
  Voltage Sensor1/RConn1 -- PS Product/LConn2
  PS Gain1/RConn1 -- PS Product/LConn1
  PS Gain1/LConn1 -- PS Product1/LConn1 -- PS Add1/LConn2 -- Simulink-PS Converter/RConn1
  PS Divide1/LConn1 -- PS Product1/RConn1
  PS Divide1/LConn2 -- PS Add1/RConn1
  PS Constant/RConn1 -- PS Add1/LConn1

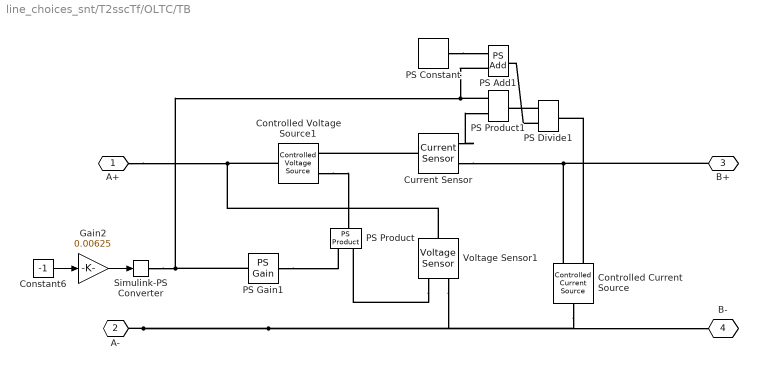
== system line_choices_snt/T2sscTf/OLTC/TB ==
  Constant6 : Constant  Value=-1
  Controlled Current Source : fl_lib/Electrical/Electrical Sources/Controlled Current Source
  Controlled Voltage Source1 : fl_lib/Electrical/Electrical Sources/Controlled Voltage Source
  Current Sensor : fl_lib/Electrical/Electrical Sensors/Current Sensor
  Gain2 : Gain  Gain=0.00625
  PS Add1 : fl_lib/Physical Signals/Functions/PS Add
  PS Constant : fl_lib/Physical Signals/Sources/PS Constant  constant=1
  PS Divide1 : fl_lib/Physical Signals/Functions/PS Divide
  PS Gain1 : fl_lib/Physical Signals/Functions/PS Gain  gain=-1
  PS Product : fl_lib/Physical Signals/Functions/PS Product
  PS Product1 : fl_lib/Physical Signals/Functions/PS Product
  Simulink-PS Converter : nesl_utility/Simulink-PS Converter  PhysicalDomain=network_engine_domain  SubClassName=ps_input  LeftPortType=input  RightPortType=output  PseudoPeriodic=off  Frequencies=[]  NoiseDistribution=none  NoiseParameters=[]  Unit=1  AffineConversion=off  FilteringAndDerivatives=zero  SimscapeFilterOrder=1  InputFilterTimeConstant=0.001  UdotUserProvided=0
  Voltage Sensor1 : fl_lib/Electrical/Electrical Sensors/Voltage Sensor
  A+ : PMIOPort  Side=Left
  A- : PMIOPort  Port=2  Side=Left
  B+ : PMIOPort  Port=3  Side=Right
  B- : PMIOPort  Port=4  Side=Right
  wires:
  Gain2/1 -> Simulink-PS Converter/1
  Constant6/1 -> Gain2/1
  connections:
  PS Constant/RConn1 -- PS Add1/LConn1
  PS Divide1/LConn2 -- PS Add1/RConn1
  PS Divide1/LConn1 -- PS Product1/RConn1
  Simulink-PS Converter/RConn1 -- PS Add1/LConn2 -- PS Product1/LConn1 -- PS Gain1/LConn1
  PS Gain1/RConn1 -- PS Product/LConn1
  Voltage Sensor1/RConn1 -- PS Product/LConn2
  A+/RConn1 -- Controlled Voltage Source1/LConn1 -- Voltage Sensor1/LConn1
  Current Sensor/LConn1 -- Controlled Voltage Source1/RConn2
  Controlled Current Source/RConn2 -- B+/RConn1 -- Current Sensor/RConn2
  A-/RConn1 -- Controlled Current Source/LConn1 -- B-/RConn1 -- Voltage Sensor1/RConn2
  Controlled Voltage Source1/RConn1 -- PS Product/RConn1
  Current Sensor/RConn1 -- PS Product1/LConn2
  Controlled Current Source/RConn1 -- PS Divide1/RConn1

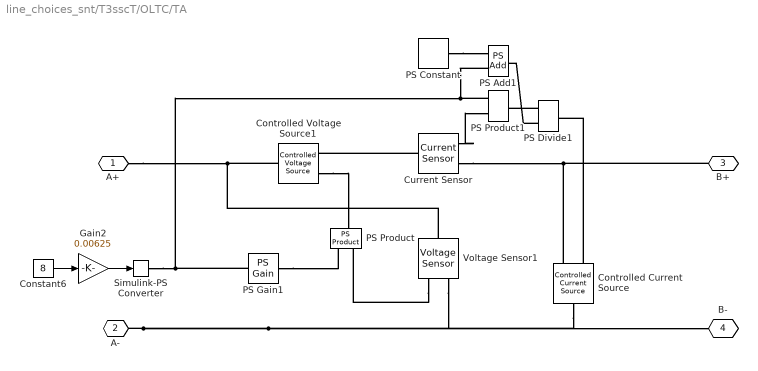
== system line_choices_snt/T3sscT/OLTC/TA ==
  Constant6 : Constant  Value=8
  Controlled Current Source : fl_lib/Electrical/Electrical Sources/Controlled Current Source
  Controlled Voltage Source1 : fl_lib/Electrical/Electrical Sources/Controlled Voltage Source
  Current Sensor : fl_lib/Electrical/Electrical Sensors/Current Sensor
  Gain2 : Gain  Gain=0.00625
  PS Add1 : fl_lib/Physical Signals/Functions/PS Add
  PS Constant : fl_lib/Physical Signals/Sources/PS Constant  constant=1
  PS Divide1 : fl_lib/Physical Signals/Functions/PS Divide
  PS Gain1 : fl_lib/Physical Signals/Functions/PS Gain  gain=-1
  PS Product : fl_lib/Physical Signals/Functions/PS Product
  PS Product1 : fl_lib/Physical Signals/Functions/PS Product
  Simulink-PS Converter : nesl_utility/Simulink-PS Converter  PhysicalDomain=network_engine_domain  SubClassName=ps_input  LeftPortType=input  RightPortType=output  PseudoPeriodic=off  Frequencies=[]  NoiseDistribution=none  NoiseParameters=[]  Unit=1  AffineConversion=off  FilteringAndDerivatives=zero  SimscapeFilterOrder=1  InputFilterTimeConstant=0.001  UdotUserProvided=0
  Voltage Sensor1 : fl_lib/Electrical/Electrical Sensors/Voltage Sensor
  A+ : PMIOPort  Side=Left
  A- : PMIOPort  Port=2  Side=Left
  B+ : PMIOPort  Port=3  Side=Right
  B- : PMIOPort  Port=4  Side=Right
  wires:
  Gain2/1 -> Simulink-PS Converter/1
  Constant6/1 -> Gain2/1
  connections:
  PS Constant/RConn1 -- PS Add1/LConn1
  PS Divide1/LConn2 -- PS Add1/RConn1
  PS Divide1/LConn1 -- PS Product1/RConn1
  Simulink-PS Converter/RConn1 -- PS Add1/LConn2 -- PS Product1/LConn1 -- PS Gain1/LConn1
  PS Gain1/RConn1 -- PS Product/LConn1
  Voltage Sensor1/RConn1 -- PS Product/LConn2
  A+/RConn1 -- Controlled Voltage Source1/LConn1 -- Voltage Sensor1/LConn1
  Current Sensor/LConn1 -- Controlled Voltage Source1/RConn2
  Controlled Current Source/RConn2 -- B+/RConn1 -- Current Sensor/RConn2
  A-/RConn1 -- Controlled Current Source/LConn1 -- B-/RConn1 -- Voltage Sensor1/RConn2
  Controlled Voltage Source1/RConn1 -- PS Product/RConn1
  Current Sensor/RConn1 -- PS Product1/LConn2
  Controlled Current Source/RConn1 -- PS Divide1/RConn1

== system line_choices_snt/T3sscT/OLTC/TB ==
  Constant6 : Constant
  Controlled Current Source : fl_lib/Electrical/Electrical Sources/Controlled Current Source
  Controlled Voltage Source1 : fl_lib/Electrical/Electrical Sources/Controlled Voltage Source
  Current Sensor : fl_lib/Electrical/Electrical Sensors/Current Sensor
  Gain2 : Gain  Gain=0.00625
  PS Add1 : fl_lib/Physical Signals/Functions/PS Add
  PS Constant : fl_lib/Physical Signals/Sources/PS Constant  constant=1
  PS Divide1 : fl_lib/Physical Signals/Functions/PS Divide
  PS Gain1 : fl_lib/Physical Signals/Functions/PS Gain  gain=-1
  PS Product : fl_lib/Physical Signals/Functions/PS Product
  PS Product1 : fl_lib/Physical Signals/Functions/PS Product
  Simulink-PS Converter : nesl_utility/Simulink-PS Converter  PhysicalDomain=network_engine_domain  SubClassName=ps_input  LeftPortType=input  RightPortType=output  PseudoPeriodic=off  Frequencies=[]  NoiseDistribution=none  NoiseParameters=[]  Unit=1  AffineConversion=off  FilteringAndDerivatives=zero  SimscapeFilterOrder=1  InputFilterTimeConstant=0.001  UdotUserProvided=0
  Voltage Sensor1 : fl_lib/Electrical/Electrical Sensors/Voltage Sensor
  A+ : PMIOPort  Side=Left
  A- : PMIOPort  Port=2  Side=Left
  B+ : PMIOPort  Port=3  Side=Right
  B- : PMIOPort  Port=4  Side=Right
  wires:
  Constant6/1 -> Gain2/1
  Gain2/1 -> Simulink-PS Converter/1
  connections:
  Controlled Current Source/RConn1 -- PS Divide1/RConn1
  Current Sensor/RConn1 -- PS Product1/LConn2
  Controlled Voltage Source1/RConn1 -- PS Product/RConn1
  Voltage Sensor1/RConn2 -- B-/RConn1 -- Controlled Current Source/LConn1 -- A-/RConn1
  Current Sensor/RConn2 -- B+/RConn1 -- Controlled Current Source/RConn2
  Current Sensor/LConn1 -- Controlled Voltage Source1/RConn2
  Voltage Sensor1/LConn1 -- Controlled Voltage Source1/LConn1 -- A+/RConn1
  Voltage Sensor1/RConn1 -- PS Product/LConn2
  PS Gain1/RConn1 -- PS Product/LConn1
  PS Gain1/LConn1 -- PS Product1/LConn1 -- PS Add1/LConn2 -- Simulink-PS Converter/RConn1
  PS Divide1/LConn1 -- PS Product1/RConn1
  PS Divide1/LConn2 -- PS Add1/RConn1
  PS Constant/RConn1 -- PS Add1/LConn1

== system line_choices_snt/T3sscT/OLTC/TC ==
  Constant6 : Constant  Value=5
  Controlled Current Source : fl_lib/Electrical/Electrical Sources/Controlled Current Source
  Controlled Voltage Source1 : fl_lib/Electrical/Electrical Sources/Controlled Voltage Source
  Current Sensor : fl_lib/Electrical/Electrical Sensors/Current Sensor
  Gain2 : Gain  Gain=0.00625
  PS Add1 : fl_lib/Physical Signals/Functions/PS Add
  PS Constant : fl_lib/Physical Signals/Sources/PS Constant  constant=1
  PS Divide1 : fl_lib/Physical Signals/Functions/PS Divide
  PS Gain1 : fl_lib/Physical Signals/Functions/PS Gain  gain=-1
  PS Product : fl_lib/Physical Signals/Functions/PS Product
  PS Product1 : fl_lib/Physical Signals/Functions/PS Product
  Simulink-PS Converter : nesl_utility/Simulink-PS Converter  PhysicalDomain=network_engine_domain  SubClassName=ps_input  LeftPortType=input  RightPortType=output  PseudoPeriodic=off  Frequencies=[]  NoiseDistribution=none  NoiseParameters=[]  Unit=1  AffineConversion=off  FilteringAndDerivatives=zero  SimscapeFilterOrder=1  InputFilterTimeConstant=0.001  UdotUserProvided=0
  Voltage Sensor1 : fl_lib/Electrical/Electrical Sensors/Voltage Sensor
  A+ : PMIOPort  Side=Left
  A- : PMIOPort  Port=2  Side=Left
  B+ : PMIOPort  Port=3  Side=Right
  B- : PMIOPort  Port=4  Side=Right
  wires:
  Gain2/1 -> Simulink-PS Converter/1
  Constant6/1 -> Gain2/1
  connections:
  PS Constant/RConn1 -- PS Add1/LConn1
  PS Divide1/LConn2 -- PS Add1/RConn1
  PS Divide1/LConn1 -- PS Product1/RConn1
  Simulink-PS Converter/RConn1 -- PS Add1/LConn2 -- PS Product1/LConn1 -- PS Gain1/LConn1
  PS Gain1/RConn1 -- PS Product/LConn1
  Voltage Sensor1/RConn1 -- PS Product/LConn2
  A+/RConn1 -- Controlled Voltage Source1/LConn1 -- Voltage Sensor1/LConn1
  Current Sensor/LConn1 -- Controlled Voltage Source1/RConn2
  Controlled Current Source/RConn2 -- B+/RConn1 -- Current Sensor/RConn2
  A-/RConn1 -- Controlled Current Source/LConn1 -- B-/RConn1 -- Voltage Sensor1/RConn2
  Controlled Voltage Source1/RConn1 -- PS Product/RConn1
  Current Sensor/RConn1 -- PS Product1/LConn2
  Controlled Current Source/RConn1 -- PS Divide1/RConn1

== system line_choices_snt/T3sscTf/OLTC/TA ==
  Constant6 : Constant  Value=8
  Controlled Current Source : fl_lib/Electrical/Electrical Sources/Controlled Current Source
  Controlled Voltage Source1 : fl_lib/Electrical/Electrical Sources/Controlled Voltage Source
  Current Sensor : fl_lib/Electrical/Electrical Sensors/Current Sensor
  Gain2 : Gain  Gain=0.00625
  PS Add1 : fl_lib/Physical Signals/Functions/PS Add
  PS Constant : fl_lib/Physical Signals/Sources/PS Constant  constant=1
  PS Divide1 : fl_lib/Physical Signals/Functions/PS Divide
  PS Gain1 : fl_lib/Physical Signals/Functions/PS Gain  gain=-1
  PS Product : fl_lib/Physical Signals/Functions/PS Product
  PS Product1 : fl_lib/Physical Signals/Functions/PS Product
  Simulink-PS Converter : nesl_utility/Simulink-PS Converter  PhysicalDomain=network_engine_domain  SubClassName=ps_input  LeftPortType=input  RightPortType=output  PseudoPeriodic=off  Frequencies=[]  NoiseDistribution=none  NoiseParameters=[]  Unit=1  AffineConversion=off  FilteringAndDerivatives=zero  SimscapeFilterOrder=1  InputFilterTimeConstant=0.001  UdotUserProvided=0
  Voltage Sensor1 : fl_lib/Electrical/Electrical Sensors/Voltage Sensor
  A+ : PMIOPort  Side=Left
  A- : PMIOPort  Port=2  Side=Left
  B+ : PMIOPort  Port=3  Side=Right
  B- : PMIOPort  Port=4  Side=Right
  wires:
  Constant6/1 -> Gain2/1
  Gain2/1 -> Simulink-PS Converter/1
  connections:
  Controlled Current Source/RConn1 -- PS Divide1/RConn1
  Current Sensor/RConn1 -- PS Product1/LConn2
  Controlled Voltage Source1/RConn1 -- PS Product/RConn1
  Voltage Sensor1/RConn2 -- B-/RConn1 -- Controlled Current Source/LConn1 -- A-/RConn1
  Current Sensor/RConn2 -- B+/RConn1 -- Controlled Current Source/RConn2
  Current Sensor/LConn1 -- Controlled Voltage Source1/RConn2
  Voltage Sensor1/LConn1 -- Controlled Voltage Source1/LConn1 -- A+/RConn1
  Voltage Sensor1/RConn1 -- PS Product/LConn2
  PS Gain1/RConn1 -- PS Product/LConn1
  PS Gain1/LConn1 -- PS Product1/LConn1 -- PS Add1/LConn2 -- Simulink-PS Converter/RConn1
  PS Divide1/LConn1 -- PS Product1/RConn1
  PS Divide1/LConn2 -- PS Add1/RConn1
  PS Constant/RConn1 -- PS Add1/LConn1

== system line_choices_snt/T3sscTf/OLTC/TB ==
  Constant6 : Constant
  Controlled Current Source : fl_lib/Electrical/Electrical Sources/Controlled Current Source
  Controlled Voltage Source1 : fl_lib/Electrical/Electrical Sources/Controlled Voltage Source
  Current Sensor : fl_lib/Electrical/Electrical Sensors/Current Sensor
  Gain2 : Gain  Gain=0.00625
  PS Add1 : fl_lib/Physical Signals/Functions/PS Add
  PS Constant : fl_lib/Physical Signals/Sources/PS Constant  constant=1
  PS Divide1 : fl_lib/Physical Signals/Functions/PS Divide
  PS Gain1 : fl_lib/Physical Signals/Functions/PS Gain  gain=-1
  PS Product : fl_lib/Physical Signals/Functions/PS Product
  PS Product1 : fl_lib/Physical Signals/Functions/PS Product
  Simulink-PS Converter : nesl_utility/Simulink-PS Converter  PhysicalDomain=network_engine_domain  SubClassName=ps_input  LeftPortType=input  RightPortType=output  PseudoPeriodic=off  Frequencies=[]  NoiseDistribution=none  NoiseParameters=[]  Unit=1  AffineConversion=off  FilteringAndDerivatives=zero  SimscapeFilterOrder=1  InputFilterTimeConstant=0.001  UdotUserProvided=0
  Voltage Sensor1 : fl_lib/Electrical/Electrical Sensors/Voltage Sensor
  A+ : PMIOPort  Side=Left
  A- : PMIOPort  Port=2  Side=Left
  B+ : PMIOPort  Port=3  Side=Right
  B- : PMIOPort  Port=4  Side=Right
  wires:
  Gain2/1 -> Simulink-PS Converter/1
  Constant6/1 -> Gain2/1
  connections:
  PS Constant/RConn1 -- PS Add1/LConn1
  PS Divide1/LConn2 -- PS Add1/RConn1
  PS Divide1/LConn1 -- PS Product1/RConn1
  Simulink-PS Converter/RConn1 -- PS Add1/LConn2 -- PS Product1/LConn1 -- PS Gain1/LConn1
  PS Gain1/RConn1 -- PS Product/LConn1
  Voltage Sensor1/RConn1 -- PS Product/LConn2
  A+/RConn1 -- Controlled Voltage Source1/LConn1 -- Voltage Sensor1/LConn1
  Current Sensor/LConn1 -- Controlled Voltage Source1/RConn2
  Controlled Current Source/RConn2 -- B+/RConn1 -- Current Sensor/RConn2
  A-/RConn1 -- Controlled Current Source/LConn1 -- B-/RConn1 -- Voltage Sensor1/RConn2
  Controlled Voltage Source1/RConn1 -- PS Product/RConn1
  Current Sensor/RConn1 -- PS Product1/LConn2
  Controlled Current Source/RConn1 -- PS Divide1/RConn1

== system line_choices_snt/T3sscTf/OLTC/TC ==
  Constant6 : Constant  Value=5
  Controlled Current Source : fl_lib/Electrical/Electrical Sources/Controlled Current Source
  Controlled Voltage Source1 : fl_lib/Electrical/Electrical Sources/Controlled Voltage Source
  Current Sensor : fl_lib/Electrical/Electrical Sensors/Current Sensor
  Gain2 : Gain  Gain=0.00625
  PS Add1 : fl_lib/Physical Signals/Functions/PS Add
  PS Constant : fl_lib/Physical Signals/Sources/PS Constant  constant=1
  PS Divide1 : fl_lib/Physical Signals/Functions/PS Divide
  PS Gain1 : fl_lib/Physical Signals/Functions/PS Gain  gain=-1
  PS Product : fl_lib/Physical Signals/Functions/PS Product
  PS Product1 : fl_lib/Physical Signals/Functions/PS Product
  Simulink-PS Converter : nesl_utility/Simulink-PS Converter  PhysicalDomain=network_engine_domain  SubClassName=ps_input  LeftPortType=input  RightPortType=output  PseudoPeriodic=off  Frequencies=[]  NoiseDistribution=none  NoiseParameters=[]  Unit=1  AffineConversion=off  FilteringAndDerivatives=zero  SimscapeFilterOrder=1  InputFilterTimeConstant=0.001  UdotUserProvided=0
  Voltage Sensor1 : fl_lib/Electrical/Electrical Sensors/Voltage Sensor
  A+ : PMIOPort  Side=Left
  A- : PMIOPort  Port=2  Side=Left
  B+ : PMIOPort  Port=3  Side=Right
  B- : PMIOPort  Port=4  Side=Right
  wires:
  Constant6/1 -> Gain2/1
  Gain2/1 -> Simulink-PS Converter/1
  connections:
  Controlled Current Source/RConn1 -- PS Divide1/RConn1
  Current Sensor/RConn1 -- PS Product1/LConn2
  Controlled Voltage Source1/RConn1 -- PS Product/RConn1
  Voltage Sensor1/RConn2 -- B-/RConn1 -- Controlled Current Source/LConn1 -- A-/RConn1
  Current Sensor/RConn2 -- B+/RConn1 -- Controlled Current Source/RConn2
  Current Sensor/LConn1 -- Controlled Voltage Source1/RConn2
  Voltage Sensor1/LConn1 -- Controlled Voltage Source1/LConn1 -- A+/RConn1
  Voltage Sensor1/RConn1 -- PS Product/LConn2
  PS Gain1/RConn1 -- PS Product/LConn1
  PS Gain1/LConn1 -- PS Product1/LConn1 -- PS Add1/LConn2 -- Simulink-PS Converter/RConn1
  PS Divide1/LConn1 -- PS Product1/RConn1
  PS Divide1/LConn2 -- PS Add1/RConn1
  PS Constant/RConn1 -- PS Add1/LConn1
